simulink model "ADC_reader_simulink"  (R2025a)
settings: Solver=FixedStepAuto  StartTime=0.0  StopTime=inf  RelTol=1e-3  EnableMultiTasking=on
libraries: stm32f4xxblockslib x7
settings Model: STM32="{\"AnalogInput\":[{\"ID\":\"test_poten:20\"},{\"ID\":\"test_poten:28\"},{\"ID\":\"ADC_reader:28\"},{\"ID\":\"ADC_reader:20\"},{\"ID\":\"ADC_reader:14\"},{\"ID\":\"ADC_reader:11\"},{\"ID\":\"ADC_reader:8\"},{\"ID\":\"ADC_reader:5\"},{\"ID\":\"ADC_reader:1\"},{\"ID\":\"ADC_reader_simulink:14\"},{\"ID\":\"ADC_reader_simulink:11\"},{\"ID\":\"ADC_reader_simulink:8\"},{\"ID\":\"ADC_reader_simulink:5\"},{\"ID\":\"ADC_reader_simulink:1\"}]}"  SimulationMode=accelerator  SnapshotInterval=1  Creator=ioonz  LastModifiedBy=ASUS
settings OptimizationCC: DefaultParameterBehavior=Inlined  EnhancedBackFolding=on  PassReuseOutputArgsAs=Individual arguments  ZeroExternalMemoryAtStartup=off  ZeroInternalMemoryAtStartup=off  MaxStackSize=512  OptimizeBlockOrder=speed  DifferentSizesBufferReuse=on  OptimizationCustomize=off  EfficientTunableParamExpr=on
settings DebuggingCC: ParameterTunabilityLossMsg=error
settings HardwareCC: ProdBitPerPointer=32.0  ProdBitPerSizeT=32.0  ProdBitPerPtrDiffT=32.0  ProdLargestAtomicInteger=Long  ProdLargestAtomicFloat=Double  ProdWordSize=32.0  ProdLongLongMode=on  ProdHWDeviceType=ARM Compatible->ARM Cortex-M
settings SFSimCC: MATLABDynamicMemAlloc=off
settings RTWCC: SystemTargetFile=ert.tlc  HardwareBoard=STM32G4xx Based  TemplateMakefile=ert_default_tmf  Toolchain=GNU Tools for ARM Embedded Processors  Description=Embedded Coder
settings CodeAppCC: ForceParamTrailComments=on  IgnoreCustomStorageClasses=off  OperatorAnnotations=on  SimulinkDataObjDesc=on  SFDataObjDesc=on  InsertBlockDesc=on
settings ERTTargetCC: ExtModeTransport=3.0  ExtModeStaticAllocSize=2048.0  TargetLangStandard=C99 (ISO)  CodeReplacementLibrary=ARM Cortex-M

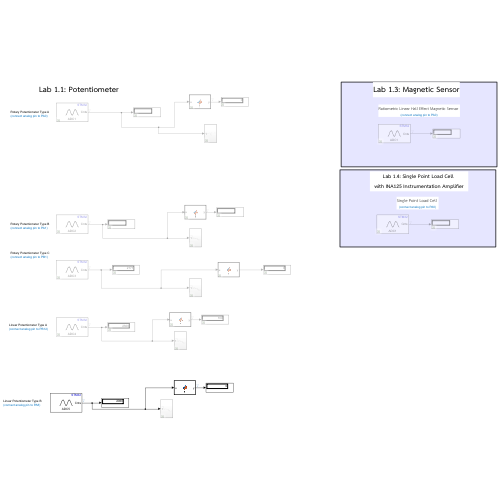
[thumbnail: Simulink's stored preview of the top-level diagram]
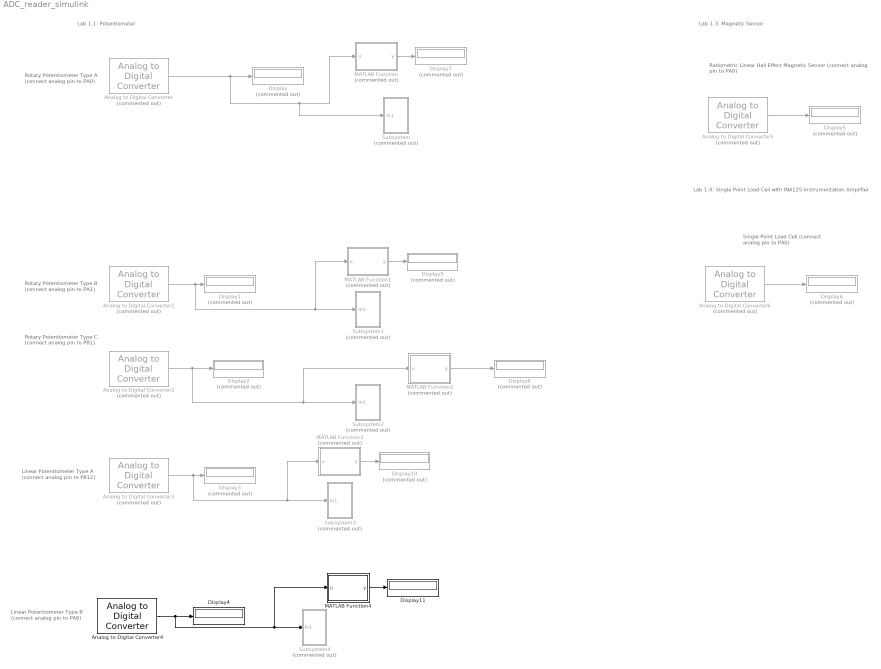
== system ADC_reader_simulink ==
  note: Lab 1.1: Potentiometer
  note: Rotary Potentiometer Type A
      | (connect analog pin to PA0)
  note: Rotary Potentiometer Type B
      | (connect analog pin to PA1)
  note: Rotary Potentiometer Type C
      | (connect analog pin to PB1)
  note: Linear Potentiometer Type A
      | (connect analog pin to PB12)
  note: Linear Potentiometer Type B
      | (connect analog pin to PA8)
  note: Ratiometric Linear Hall Effect Magnetic Sensor
      | (connect analog pin to PA0)
  note: Single Point Load Cell
      | (connect analog pin to PA0)
  note: Lab 1.3: Magnetic Sensor
  note: Lab 1.4: Single Point Load Cell
      | with INA125 Instrumentation Amplifier
  Analog to Digital Converter : stm32f4xxblockslib/Analog to Digital Converter  Commented=on  ADCModule=ADC1  ConversionGroup=Regular  TriggerMode=Trigger and read  NumberOfConversions=1  EnableBufferConv=off  BufferLength=1  OutputStatus=off  SampleTime=-1  EnableSimPort=off  hoistedMaskSrc=ECSoC/ECSimCodegen/Analog to Digital Converter
  Analog to Digital Converter1 : stm32f4xxblockslib/Analog to Digital Converter  Commented=on  ADCModule=ADC2  ConversionGroup=Regular  TriggerMode=Trigger and read  NumberOfConversions=1  EnableBufferConv=off  BufferLength=1  OutputStatus=off  SampleTime=-1  EnableSimPort=off  hoistedMaskSrc=ECSoC/ECSimCodegen/Analog to Digital Converter
  Analog to Digital Converter2 : stm32f4xxblockslib/Analog to Digital Converter  Commented=on  ADCModule=ADC3  ConversionGroup=Regular  TriggerMode=Trigger and read  NumberOfConversions=1  EnableBufferConv=off  BufferLength=1  OutputStatus=off  SampleTime=-1  EnableSimPort=off  hoistedMaskSrc=ECSoC/ECSimCodegen/Analog to Digital Converter
  Analog to Digital Converter3 : stm32f4xxblockslib/Analog to Digital Converter  Commented=on  ADCModule=ADC4  ConversionGroup=Regular  TriggerMode=Trigger and read  NumberOfConversions=1  EnableBufferConv=off  BufferLength=1  OutputStatus=off  SampleTime=-1  EnableSimPort=off  hoistedMaskSrc=ECSoC/ECSimCodegen/Analog to Digital Converter
  Analog to Digital Converter4 : stm32f4xxblockslib/Analog to Digital Converter  ADCModule=ADC5  ConversionGroup=Regular  TriggerMode=Trigger and read  NumberOfConversions=1  EnableBufferConv=off  BufferLength=1  OutputStatus=off  SampleTime=-1  EnableSimPort=off  hoistedMaskSrc=ECSoC/ECSimCodegen/Analog to Digital Converter
  Analog to Digital Converter5 : stm32f4xxblockslib/Analog to Digital Converter  Commented=on  ADCModule=ADC1  ConversionGroup=Regular  TriggerMode=Trigger and read  NumberOfConversions=1  EnableBufferConv=off  BufferLength=1  OutputStatus=off  SampleTime=-1  EnableSimPort=off  hoistedMaskSrc=ECSoC/ECSimCodegen/Analog to Digital Converter
  Analog to Digital Converter6 : stm32f4xxblockslib/Analog to Digital Converter  Commented=on  ADCModule=ADC1  ConversionGroup=Regular  TriggerMode=Trigger and read  NumberOfConversions=1  EnableBufferConv=off  BufferLength=1  OutputStatus=off  SampleTime=-1  EnableSimPort=off  hoistedMaskSrc=ECSoC/ECSimCodegen/Analog to Digital Converter
  Display{,1..3,5..10} (10 alike) : Display  Commented=on
  Display11 : Display
  Display4 : Display
  MATLAB Function : MATLAB Function  Commented=on  TreatAsAtomicUnit=on
  MATLAB Function1 : MATLAB Function  Commented=on  TreatAsAtomicUnit=on
  MATLAB Function2 : MATLAB Function  Commented=on  TreatAsAtomicUnit=on
  MATLAB Function3 : MATLAB Function  Commented=on  TreatAsAtomicUnit=on
  MATLAB Function4 : MATLAB Function  TreatAsAtomicUnit=on
  Subsystem : Subsystem  Commented=on
  Subsystem1 : Subsystem  Commented=on
  Subsystem2 : Subsystem  Commented=on
  Subsystem3 : Subsystem  Commented=on
  Subsystem4 : Subsystem  Commented=on
  wires:
  Analog to Digital Converter5/1 -> Display5/1
  Analog to Digital Converter6/1 -> Display6/1
  MATLAB Function/1(y) -> Display7/1
  Analog to Digital Converter/1 -> Subsystem/1(In1), MATLAB Function/1(u), Display/1
  MATLAB Function2/1(y) -> Display8/1
  Analog to Digital Converter2/1 -> MATLAB Function2/1(u), Subsystem2/1(In1), Display2/1
  MATLAB Function1/1(y) -> Display9/1
  Analog to Digital Converter1/1 -> MATLAB Function1/1(u), Subsystem1/1(In1), Display1/1
  MATLAB Function3/1(y) -> Display10/1
  Analog to Digital Converter3/1 -> MATLAB Function3/1(u), Subsystem3/1(In1), Display3/1
  MATLAB Function4/1(y) -> Display11/1
  Analog to Digital Converter4/1 -> MATLAB Function4/1(u), Subsystem4/1(In1), Display4/1

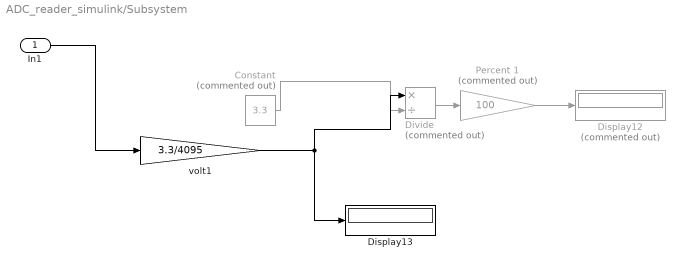
== system ADC_reader_simulink/Subsystem ==
  In1 : Inport
  Constant : Constant  Commented=on  Value=3.3
  Display12 : Display  Commented=on
  Display13 : Display
  Divide : Product  Commented=on  Inputs=*/
  Percent 1 : Gain  Commented=on  Gain=100
  volt1 : Gain  Gain=3.3/4095
  wires:
  In1/1 -> volt1/1
  Constant/1 -> Divide/2
  volt1/1 -> Divide/1, Display13/1
  Divide/1 -> Percent 1/1
  Percent 1/1 -> Display12/1

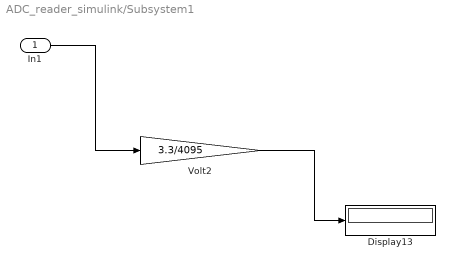
== system ADC_reader_simulink/Subsystem1 ==
  In1 : Inport
  Display13 : Display
  Volt2 : Gain  Gain=3.3/4095
  wires:
  In1/1 -> Volt2/1
  Volt2/1 -> Display13/1

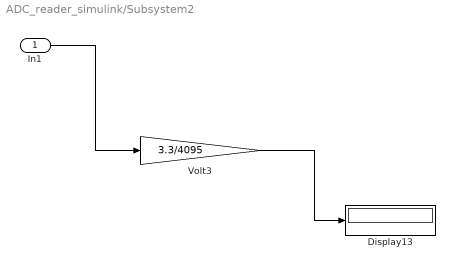
== system ADC_reader_simulink/Subsystem2 ==
  In1 : Inport
  Display13 : Display
  Volt3 : Gain  Gain=3.3/4095
  wires:
  In1/1 -> Volt3/1
  Volt3/1 -> Display13/1

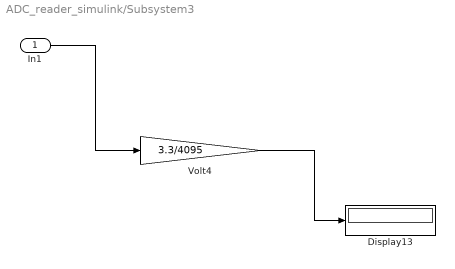
== system ADC_reader_simulink/Subsystem3 ==
  In1 : Inport
  Display13 : Display
  Volt4 : Gain  Gain=3.3/4095
  wires:
  In1/1 -> Volt4/1
  Volt4/1 -> Display13/1

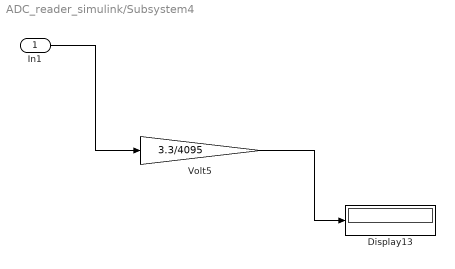
== system ADC_reader_simulink/Subsystem4 ==
  In1 : Inport
  Display13 : Display
  Volt5 : Gain  Gain=3.3/4095
  wires:
  In1/1 -> Volt5/1
  Volt5/1 -> Display13/1

== matlab function ADC_reader_simulink/MATLAB Function ==
  data: u input; y output
function y = f(u)
    
    % 1. ประกาศตัวแปร 'persistent' เพื่อให้มัน "จำ" สถานะก่อนหน้าได้
    persistent previousState;
    
    % 2. ตรวจสอบและตั้งค่าเริ่มต้น (ถ้าเป็นการรันครั้งแรก)
    if isempty(previousState)
        previousState = 0; % สมมติว่าเริ่มที่ 0
    end
    
    % 3. ตรรกะ Schmitt Trigger
    if u > 3000
        y = 100;
    elseif u < 1000
        y = 0;
    else
        % ถ้าค่าอยู่ระหว่าง 1000 ถึง 3000 (Hysteresis)
        % -> y จะคงค่าเดิมไว้
        y = previousState;
    end  % <--- ✅ นี่คือจุดที่แก้ไขแล้ว (MUST BE 'end')

    % 4. อัปเดตสถานะ "จำ" ค่า y ล่าสุดไว้สำหรับรอบถัดไป
    previousState = y;
end

== matlab function ADC_reader_simulink/MATLAB Function1 ==
  data: u input; y output
function y = f(u)
    
    % 1. ประกาศตัวแปร 'persistent' เพื่อให้มัน "จำ" สถานะก่อนหน้าได้
    persistent previousState;
    
    % 2. ตรวจสอบและตั้งค่าเริ่มต้น (ถ้าเป็นการรันครั้งแรก)
    if isempty(previousState)
        previousState = 0; % สมมติว่าเริ่มที่ 0
    end
    
    % 3. ตรรกะ Schmitt Trigger
    if u > 3000
        y = 100;
    elseif u < 1000
        y = 0;
    else
        % ถ้าค่าอยู่ระหว่าง 1000 ถึง 3000 (Hysteresis)
        % -> y จะคงค่าเดิมไว้
        y = previousState;
    end  % <--- ✅ นี่คือจุดที่แก้ไขแล้ว (MUST BE 'end')

    % 4. อัปเดตสถานะ "จำ" ค่า y ล่าสุดไว้สำหรับรอบถัดไป
    previousState = y;
end

== matlab function ADC_reader_simulink/MATLAB Function3 ==
  data: u input; y output
function y = f(u)
    
    % 1. ประกาศตัวแปร 'persistent' เพื่อให้มัน "จำ" สถานะก่อนหน้าได้
    persistent previousState;
    
    % 2. ตรวจสอบและตั้งค่าเริ่มต้น (ถ้าเป็นการรันครั้งแรก)
    if isempty(previousState)
        previousState = 0; % สมมติว่าเริ่มที่ 0
    end
    
    % 3. ตรรกะ Schmitt Trigger
    if u > 3000
        y = 100;
    elseif u < 1000
        y = 0;
    else
        % ถ้าค่าอยู่ระหว่าง 1000 ถึง 3000 (Hysteresis)
        % -> y จะคงค่าเดิมไว้
        y = previousState;
    end  % <--- ✅ นี่คือจุดที่แก้ไขแล้ว (MUST BE 'end')

    % 4. อัปเดตสถานะ "จำ" ค่า y ล่าสุดไว้สำหรับรอบถัดไป
    previousState = y;
end

== matlab function ADC_reader_simulink/MATLAB Function4 ==
  data: u input; y output
function y = f(u)
    
    % 1. ประกาศตัวแปร 'persistent' เพื่อให้มัน "จำ" สถานะก่อนหน้าได้
    persistent previousState;
    
    % 2. ตรวจสอบและตั้งค่าเริ่มต้น (ถ้าเป็นการรันครั้งแรก)
    if isempty(previousState)
        previousState = 0; % สมมติว่าเริ่มที่ 0
    end
    
    % 3. ตรรกะ Schmitt Trigger
    if u > 3000
        y = 100;
    elseif u < 1000
        y = 0;
    else
        % ถ้าค่าอยู่ระหว่าง 1000 ถึง 3000 (Hysteresis)
        % -> y จะคงค่าเดิมไว้
        y = previousState;
    end  % <--- ✅ นี่คือจุดที่แก้ไขแล้ว (MUST BE 'end')

    % 4. อัปเดตสถานะ "จำ" ค่า y ล่าสุดไว้สำหรับรอบถัดไป
    previousState = y;
end

== matlab function ADC_reader_simulink/MATLAB Function2 ==
  data: u input; y output
function y = f(u)
    
    % 1. ประกาศตัวแปร 'persistent' เพื่อให้มัน "จำ" สถานะก่อนหน้าได้
    persistent previousState;
    
    % 2. ตรวจสอบและตั้งค่าเริ่มต้น (ถ้าเป็นการรันครั้งแรก)
    if isempty(previousState)
        previousState = 0; % สมมติว่าเริ่มที่ 0
    end
    
    % 3. ตรรกะ Schmitt Trigger
    if u > 3000
        y = 100;
    elseif u < 1000
        y = 0;
    else
        % ถ้าค่าอยู่ระหว่าง 1000 ถึง 3000 (Hysteresis)
        % -> y จะคงค่าเดิมไว้
        y = previousState;
    end  % <--- ✅ นี่คือจุดที่แก้ไขแล้ว (MUST BE 'end')

    % 4. อัปเดตสถานะ "จำ" ค่า y ล่าสุดไว้สำหรับรอบถัดไป
    previousState = y;
end
